simulink model "xy_eqn_model"  (R2022a)
settings: Solver=ode45  StartTime=0.0  StopTime=1  RelTol=1e-7
settings Model: Creator=Sukruth  LastModifiedBy=Sukruth

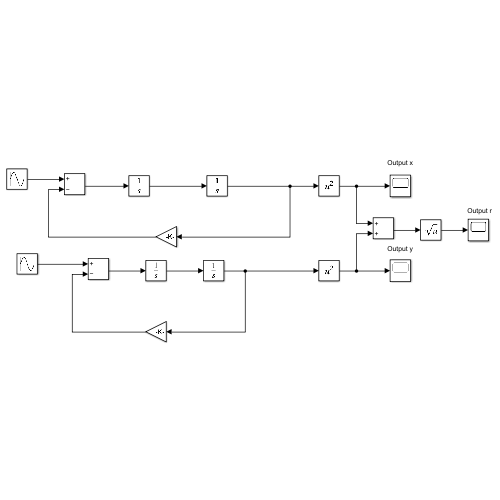
[thumbnail: Simulink's stored preview of the top-level diagram]
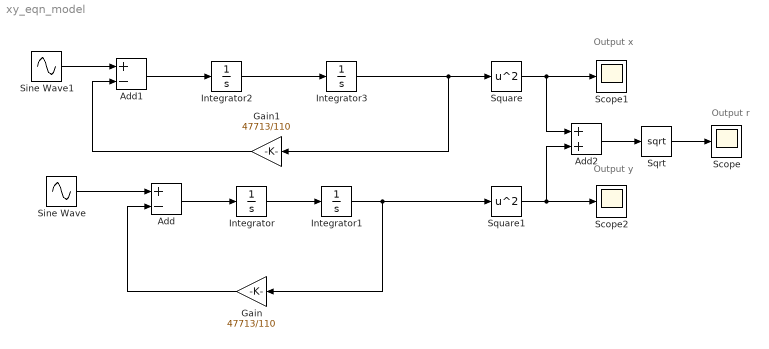
== system xy_eqn_model ==
  note: Output y
  note: Output x
  note: Output r
  Add : Sum  Inputs=+-
  Add1 : Sum  Inputs=+-
  Add2 : Sum
  Gain : Gain  Gain=47713/110
  Gain1 : Gain  Gain=47713/110
  Integrator{,1..3} (4 alike) : Integrator
  Scope : Scope
  Scope1 : Scope
  Scope2 : Scope
  Sine Wave : Sin  Amplitude=0.075*37.699*37.699  Frequency=37.699  SampleTime=0
  Sine Wave1 : Sin  Amplitude=0.075*37.699*37.699  Frequency=37.699  Phase=pi/2  SampleTime=0
  Sqrt : Sqrt
  Square : Math  Operator=square
  Square1 : Math  Operator=square
  wires:
  Sine Wave/1 -> Add/1
  Integrator/1 -> Integrator1/1
  Gain/1 -> Add/2
  Add/1 -> Integrator/1
  Sine Wave1/1 -> Add1/1
  Add1/1 -> Integrator2/1
  Integrator2/1 -> Integrator3/1
  Gain1/1 -> Add1/2
  Integrator3/1 -> Square/1, Gain1/1
  Integrator1/1 -> Square1/1, Gain/1
  Square/1 -> Scope1/1, Add2/1
  Add2/1 -> Sqrt/1
  Sqrt/1 -> Scope/1
  Square1/1 -> Add2/2, Scope2/1
